simulink model "Res_6"  (R2018b)
settings: Solver=VariableStepAuto  StartTime=0.0  StopTime=2  RelTol=1e-3
settings Model: Creator=makha  LastModifiedBy=makha

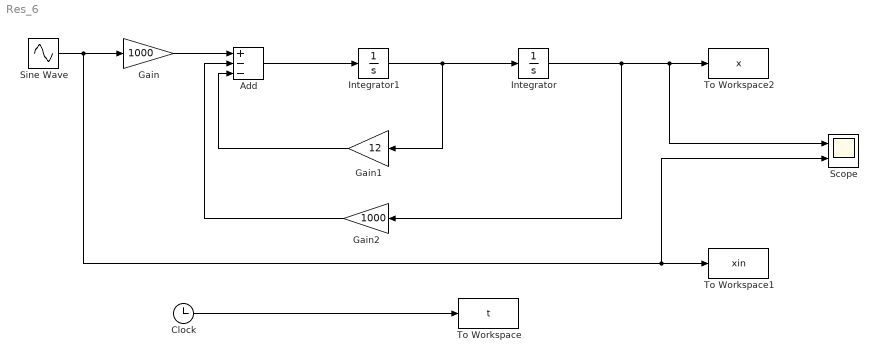
== system Res_6 ==
  Add : Sum  Inputs=+--
  Clock : Clock
  Gain : Gain  Gain=1000
  Gain1 : Gain  Gain=12
  Gain2 : Gain  Gain=1000
  Integrator : Integrator
  Integrator1 : Integrator
  Scope : Scope  NumInputPorts=2
  Sine Wave : Sin  Amplitude=0.05  Frequency=20  SampleTime=0.0001
  To Workspace : ToWorkspace  VariableName=t  SampleTime=-1
  To Workspace1 : ToWorkspace  VariableName=xin  SampleTime=-1
  To Workspace2 : ToWorkspace  VariableName=x  SampleTime=-1
  wires:
  Sine Wave/1 -> Gain/1, Scope/2, To Workspace1/1
  Gain/1 -> Add/1
  Add/1 -> Integrator1/1
  Integrator1/1 -> Gain1/1, Integrator/1
  Clock/1 -> To Workspace/1
  Gain1/1 -> Add/3
  Gain2/1 -> Add/2
  Integrator/1 -> Gain2/1, Scope/1, To Workspace2/1
